simulink model "innerControllerTuning4"  (R2018a)
settings: Solver=VariableStepAuto  StartTime=0.0  StopTime=10  RelTol=1e-3
values from neighbouring files (symbols this model uses):
  d = 2.4*10^-3    (= 0.0024)    [innerInit.m]    (also in outerInit.m)
  g = 9.81    [innerInit.m]    (also in outerInit.m)
  Ixx = 5.9*10^-3    (= 0.0059)    [innerInit.m]    (also in outerInit.m)
  Iyy = 5.9*10^-3    (= 0.0059)    [innerInit.m]    (also in outerInit.m)
  Izz = 1.16*10^-3    (= 0.00116)    [innerInit.m]    (also in outerInit.m)
  kr = 0.1    [innerInit.m]    (also in outerInit.m)
  kt = 0.1    [innerInit.m]    (also in outerInit.m)
  l = 0.255    [innerInit.m]    (also in outerInit.m)
  m = 0.5    [innerInit.m]    (also in outerInit.m)
  p0 = 0.5    [innerInit.m]
  phi0 = pi/4    (= 0.785398163397)    [innerInit.m]
  q0 = 0.5    [innerInit.m]
  r0 = 2.7    [innerInit.m]
  theta0 = pi/4    (= 0.785398163397)    [innerInit.m]
libraries: simulink x2, aerolibutil x1
settings Model: Creator=giuseppe  LastModifiedBy=giuseppe

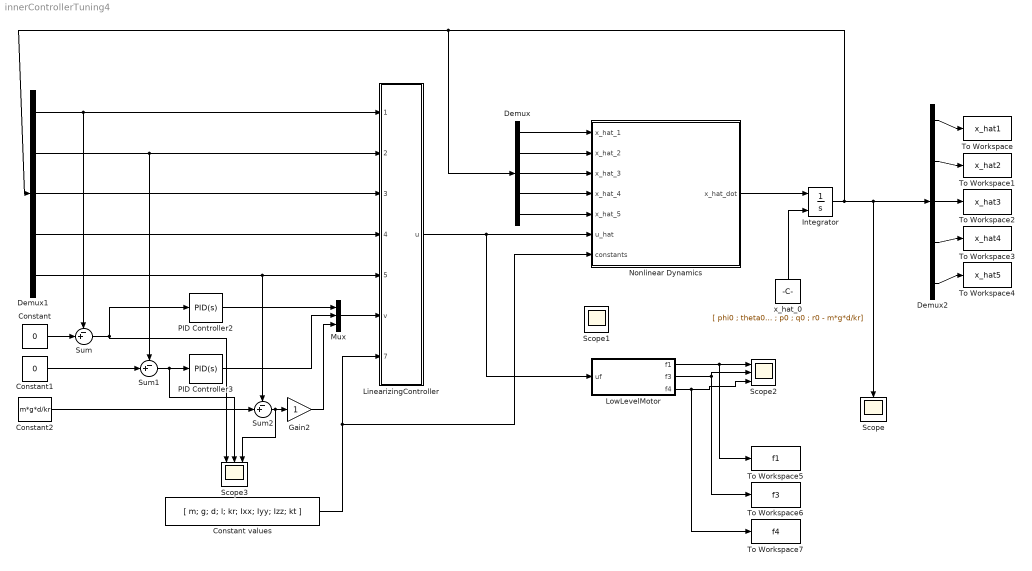
== system innerControllerTuning4 ==
  Constant : Constant  Value=0
  Constant values : Constant  Value=[ m; g; d; l; kr; Ixx; Iyy; Izz; kt ]
  Constant1 : Constant  Value=0
  Constant2 : Constant  Value=m*g*d/kr
  Demux : Demux  Outputs=5
  Demux1 : Demux  Outputs=5
  Demux2 : Demux  Outputs=5
  Gain2 : Gain
  Integrator : Integrator  InitialConditionSource=external
  LinearizingController : MATLAB Function  TreatAsAtomicUnit=on
  LowLevelMotor : Subsystem
  Mux : Mux  Inputs=3
  "Nonlinear Dynamics " : MATLAB Function  TreatAsAtomicUnit=on
  PID Controller2 : simulink/Continuous/PID Controller  Controller=PID  TimeDomain=Continuous-time  SampleTime=-1  IntegratorMethod=Forward Euler  FilterMethod=Forward Euler  Form=Parallel  UseFilter=on  ControllerParametersSource=internal  P=5  I=1  D=2  N=100  InitialConditionSource=internal  InitialConditionForIntegrator=0  InitialConditionForFilter=0  ExternalReset=none  LimitOutput=off  UpperSaturationLimit=inf  LowerSaturationLimit=-inf  LinearizeAsGain=on  AntiWindupMode=none  Kb=1  TrackingMode=off  Kt=1  PParamMin=[]  PParamMax=[]  IParamMin=[]  IParamMax=[]  DParamMin=[]  DParamMax=[]  NParamMin=[]  NParamMax=[]  KbParamMin=[]  KbParamMax=[]  KtParamMin=[]  KtParamMax=[]  POutMin=[]  POutMax=[]  IOutMin=[]  IOutMax=[]  DOutMin=[]  DOutMax=[]  NOutMin=[]  NOutMax=[]  KbOutMin=[]  KbOutMax=[]  KtOutMin=[]  KtOutMax=[]  IntegratorOutMin=[]  IntegratorOutMax=[]  FilterOutMin=[]  FilterOutMax=[]  SumOutMin=[]  SumOutMax=[]  SumI1OutMin=[]  SumI1OutMax=[]  SumI2OutMin=[]  SumI2OutMax=[]  SumI3OutMin=[]  SumI3OutMax=[]  SumDOutMin=[]  SumDOutMax=[]  SaturationOutMin=[]  SaturationOutMax=[]  IntegratorContinuousStateAttributes=''  IntegratorStateMustResolveToSignalObject=off  IntegratorRTWStateStorageClass=Auto  FilterContinuousStateAttributes=''  FilterStateMustResolveToSignalObject=off  FilterRTWStateStorageClass=Auto  DifferentiatorICPrevScaledInput=0  DifferentiatorOutMin=[]  DifferentiatorOutMax=[]  FilterDiffOutCoefMin=[]  FilterDiffOutCoefMax=[]  SumDenOutMin=[]  SumDenOutMax=[]  SumNumOutMin=[]  SumNumOutMax=[]  ReciprocalOutMin=[]  ReciprocalOutMax=[]  DivideOutMin=[]  DivideOutMax=[]  TunerSelectOption=Transfer Function Based (PID Tuner App)
  PID Controller3 : simulink/Continuous/PID Controller  Controller=PID  TimeDomain=Continuous-time  SampleTime=-1  IntegratorMethod=Forward Euler  FilterMethod=Forward Euler  Form=Parallel  UseFilter=on  ControllerParametersSource=internal  P=5  I=1  D=2  N=100  InitialConditionSource=internal  InitialConditionForIntegrator=0  InitialConditionForFilter=0  ExternalReset=none  LimitOutput=off  UpperSaturationLimit=inf  LowerSaturationLimit=-inf  LinearizeAsGain=on  AntiWindupMode=none  Kb=1  TrackingMode=off  Kt=1  PParamMin=[]  PParamMax=[]  IParamMin=[]  IParamMax=[]  DParamMin=[]  DParamMax=[]  NParamMin=[]  NParamMax=[]  KbParamMin=[]  KbParamMax=[]  KtParamMin=[]  KtParamMax=[]  POutMin=[]  POutMax=[]  IOutMin=[]  IOutMax=[]  DOutMin=[]  DOutMax=[]  NOutMin=[]  NOutMax=[]  KbOutMin=[]  KbOutMax=[]  KtOutMin=[]  KtOutMax=[]  IntegratorOutMin=[]  IntegratorOutMax=[]  FilterOutMin=[]  FilterOutMax=[]  SumOutMin=[]  SumOutMax=[]  SumI1OutMin=[]  SumI1OutMax=[]  SumI2OutMin=[]  SumI2OutMax=[]  SumI3OutMin=[]  SumI3OutMax=[]  SumDOutMin=[]  SumDOutMax=[]  SaturationOutMin=[]  SaturationOutMax=[]  IntegratorContinuousStateAttributes=''  IntegratorStateMustResolveToSignalObject=off  IntegratorRTWStateStorageClass=Auto  FilterContinuousStateAttributes=''  FilterStateMustResolveToSignalObject=off  FilterRTWStateStorageClass=Auto  DifferentiatorICPrevScaledInput=0  DifferentiatorOutMin=[]  DifferentiatorOutMax=[]  FilterDiffOutCoefMin=[]  FilterDiffOutCoefMax=[]  SumDenOutMin=[]  SumDenOutMax=[]  SumNumOutMin=[]  SumNumOutMax=[]  ReciprocalOutMin=[]  ReciprocalOutMax=[]  DivideOutMin=[]  DivideOutMax=[]  TunerSelectOption=Transfer Function Based (PID Tuner App)
  Scope : Scope
  Scope1 : Scope
  Scope2 : Scope  NumInputPorts=3
  Scope3 : Scope  NumInputPorts=3
  Sum : Sum  Inputs=-+|
  Sum1 : Sum  Inputs=-+|
  Sum2 : Sum  Inputs=-+|
  To Workspace : ToWorkspace  VariableName=x_hat1  SaveFormat=Timeseries  SampleTime=-1
  To Workspace1 : ToWorkspace  VariableName=x_hat2  SaveFormat=Timeseries  SampleTime=-1
  To Workspace2 : ToWorkspace  VariableName=x_hat3  SaveFormat=Timeseries  SampleTime=-1
  To Workspace3 : ToWorkspace  VariableName=x_hat4  SaveFormat=Timeseries  SampleTime=-1
  To Workspace4 : ToWorkspace  VariableName=x_hat5  SaveFormat=Timeseries  SampleTime=-1
  To Workspace5 : ToWorkspace  VariableName=f1  SaveFormat=Timeseries  SampleTime=-1
  To Workspace6 : ToWorkspace  VariableName=f3  SaveFormat=Timeseries  SampleTime=-1
  To Workspace7 : ToWorkspace  VariableName=f4  SaveFormat=Timeseries  SampleTime=-1
  x_hat_0 : Constant  Value=[ phi0 ; theta0 ; p0 ; q0 ; r0 - m*g*d/kr]
  wires:
  LinearizingController/1(u) -> LowLevelMotor/1(uf), "Nonlinear Dynamics "/6(u_hat)
  Constant values/1 -> "Nonlinear Dynamics "/7(constants), LinearizingController/7(constants)
  "Nonlinear Dynamics "/1(x_hat_dot) -> Integrator/1
  x_hat_0/1 -> Integrator/2
  Demux/1 -> "Nonlinear Dynamics "/1(x_hat_1)
  Demux/2 -> "Nonlinear Dynamics "/2(x_hat_2)
  Demux/3 -> "Nonlinear Dynamics "/3(x_hat_3)
  Demux/4 -> "Nonlinear Dynamics "/4(x_hat_4)
  Demux/5 -> "Nonlinear Dynamics "/5(x_hat_5)
  Integrator/1 -> Demux1/1, Demux/1, Demux2/1, Scope/1
  Demux1/5 -> LinearizingController/5(x5_hat), Sum2/1
  Demux1/4 -> LinearizingController/4(x4_hat)
  Demux1/3 -> LinearizingController/3(x3_hat)
  Demux1/2 -> Sum1/1, LinearizingController/2(x2_hat)
  Demux1/1 -> Sum/1, LinearizingController/1(x1_hat)
  Constant/1 -> Sum/2
  Constant1/1 -> Sum1/2
  Constant2/1 -> Sum2/2
  Mux/1 -> LinearizingController/6(v)
  Sum/1 -> PID Controller2/1, Scope3/1
  Sum2/1 -> Scope3/3, Gain2/1
  Gain2/1 -> Mux/3
  Sum1/1 -> PID Controller3/1, Scope3/2
  Demux2/5 -> To Workspace4/1
  Demux2/4 -> To Workspace3/1
  Demux2/3 -> To Workspace2/1
  Demux2/2 -> To Workspace1/1
  Demux2/1 -> To Workspace/1
  LowLevelMotor/3(f4) -> To Workspace7/1, Scope2/3
  LowLevelMotor/1(f1) -> To Workspace5/1, Scope2/1
  LowLevelMotor/2(f3) -> To Workspace6/1, Scope2/2
  PID Controller2/1 -> Mux/1
  PID Controller3/1 -> Mux/2

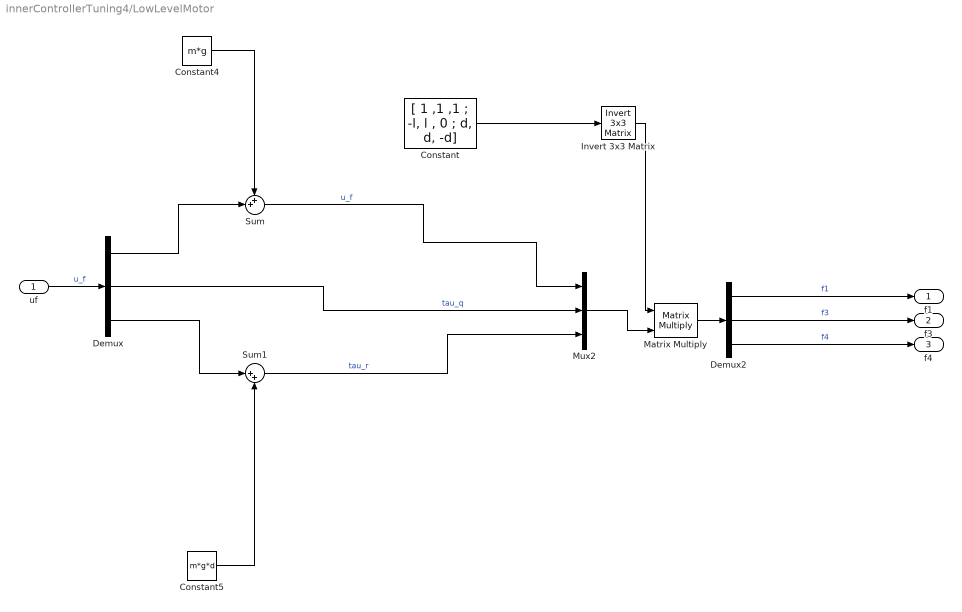
== system innerControllerTuning4/LowLevelMotor ==
  uf : Inport
  Constant : Constant  Value=[ 1 ,1 ,1 ; -l, l , 0 ; d, d, -d]
  Constant4 : Constant  Value=m*g
  Constant5 : Constant  Value=m*g*d
  Demux : Demux  Outputs=3
  Demux2 : Demux  Outputs=3
  Invert 3x3 Matrix : aerolibutil/Invert  3x3 Matrix
  Matrix Multiply : Product  Multiplication=Matrix(*)
  Mux2 : Mux  Inputs=3
  Sum : Sum  Inputs=++|
  Sum1 : Sum  Inputs=|++
  f1 : Outport
  f3 : Outport  Port=2
  f4 : Outport  Port=3
  wires:
  Demux/2 -> Mux2/2  "tau_q"
  Invert 3x3 Matrix/1 -> Matrix Multiply/1
  Sum1/1 -> Mux2/3  "tau_r"
  Mux2/1 -> Matrix Multiply/2
  Matrix Multiply/1 -> Demux2/1
  Sum/1 -> Mux2/1  "u_f"
  Constant/1 -> Invert 3x3 Matrix/1
  uf/1 -> Demux/1  "u_f"
  Constant4/1 -> Sum/1
  Demux/1 -> Sum/2
  Demux/3 -> Sum1/1
  Constant5/1 -> Sum1/2
  Demux2/1 -> f1/1  "f1"
  Demux2/2 -> f3/1  "f3"
  Demux2/3 -> f4/1  "f4"

== matlab function innerControllerTuning4/LinearizingController ==
  data: x1_hat input; u output; x2_hat input; x3_hat input; x4_hat input; x5_hat input; v input; constants input
function u = fcn(x1_hat,x2_hat,x3_hat,x4_hat,x5_hat, v, constants)

m= constants(1,1);
g= constants(2,1);
d= constants(3,1);
l= constants(4,1);
kr= constants(5,1);
Ixx= constants(6,1)
Iyy= constants(7,1);
Izz= constants(8,1);

alfa = zeros(3,1);

%% Non-robust feedback-linearation

alfa(1,1) = (2*Ixx*((kr*x3_hat - x4_hat*(x5_hat + (d*g*m)/kr)*(Ixx - Izz))/Ixx + (sin(x1_hat)*tan(x2_hat)*(x5_hat + (d*g*m)/kr) - x4_hat*cos(x1_hat)*tan(x2_hat))*(x3_hat + cos(x1_hat)*tan(x2_hat)*(x5_hat + (d*g*m)/kr) + x4_hat*sin(x1_hat)*tan(x2_hat)) + (sin(x1_hat)*(x5_hat + (d*g*m)/kr) - x4_hat*cos(x1_hat))*(cos(x1_hat)*(x5_hat + (d*g*m)/kr)*(tan(x2_hat)^2 + 1) + x4_hat*sin(x1_hat)*(tan(x2_hat)^2 + 1)) + (sin(x1_hat)*tan(x2_hat)*(kr*x4_hat + x3_hat*(x5_hat + (d*g*m)/kr)*(Ixx - Izz)))/Ixx + (kr*x5_hat*cos(x1_hat)*tan(x2_hat))/Izz))/l - (2*Ixx*sin(x1_hat)*tan(x2_hat)*((cos(x1_hat)*(x5_hat + (d*g*m)/kr) + x4_hat*sin(x1_hat))*(x3_hat + cos(x1_hat)*tan(x2_hat)*(x5_hat + (d*g*m)/kr) + x4_hat*sin(x1_hat)*tan(x2_hat)) + (cos(x1_hat)*(kr*x4_hat + x3_hat*(x5_hat + (d*g*m)/kr)*(Ixx - Izz)))/Ixx - (kr*x5_hat*sin(x1_hat))/Izz))/(l*cos(x1_hat)) - (kr*x5_hat*(2*Ixx*d*cos(x1_hat)^2*tan(x2_hat) - Izz*l*cos(x1_hat) + 2*Ixx*d*sin(x1_hat)^2*tan(x2_hat)))/(Izz*d*l*cos(x1_hat));
alfa(2,1) = (Ixx*((cos(x1_hat)*(x5_hat + (d*g*m)/kr) + x4_hat*sin(x1_hat))*(x3_hat + cos(x1_hat)*tan(x2_hat)*(x5_hat + (d*g*m)/kr) + x4_hat*sin(x1_hat)*tan(x2_hat)) + (cos(x1_hat)*(kr*x4_hat + x3_hat*(x5_hat + (d*g*m)/kr)*(Ixx - Izz)))/Ixx - (kr*x5_hat*sin(x1_hat))/Izz))/cos(x1_hat) + (Ixx*kr*x5_hat*sin(x1_hat))/(Izz*cos(x1_hat));
alfa(3,1) = kr*x5_hat;

beta =  [
         (2*Ixx)/l, -(2*Ixx*sin(x1_hat)*sin(x2_hat))/(l*cos(x1_hat)*cos(x2_hat)), -(2*Ixx*d*sin(x2_hat)-Izz*l*cos(x1_hat)*cos(x2_hat))/(d*l*cos(x1_hat)*cos(x2_hat));
         0,                                              Ixx/cos(x1_hat),                                                        (Ixx*sin(x1_hat))/cos(x1_hat);
         0,                                                            0,                                                                                  Izz];

%% Robust feedback linearization

% alfa(1,1) = x1_hat*((d*g*m*((2*Ixx*((d*g*m)/kr + (d*g*m*(Ixx - Izz))/(Ixx*kr)))/l + (2*kr*sin(x1_hat)*tan(x2_hat))/(l*cos(x1_hat))))/kr - (2*Ixx*d^2*g^2*m^2)/(kr^2*l)) - (sin(x1_hat)*(x5_hat + (d*g*m)/kr) - x4_hat*cos(x1_hat))*((2*Ixx*((d*g*m)/kr + (d*g*m*(Ixx - Izz))/(Ixx*kr)))/l + (2*kr*sin(x1_hat)*tan(x2_hat))/(l*cos(x1_hat))) + x2_hat*((d*g*m*((2*kr)/l - (2*Ixx*sin(x1_hat)*tan(x2_hat)*((d*g*m)/kr + (d*g*m*(Ixx - Izz))/(Ixx*kr)))/(l*cos(x1_hat))))/kr + (2*Ixx*d^2*g^2*m^2*sin(x1_hat)*tan(x2_hat))/(kr^2*l*cos(x1_hat))) - ((2*kr)/l - (2*Ixx*sin(x1_hat)*tan(x2_hat)*((d*g*m)/kr + (d*g*m*(Ixx - Izz))/(Ixx*kr)))/(l*cos(x1_hat)))*(x3_hat + cos(x1_hat)*tan(x2_hat)*(x5_hat + (d*g*m)/kr) + x4_hat*sin(x1_hat)*tan(x2_hat)) + (2*Ixx*((kr*x3_hat - x4_hat*(x5_hat + (d*g*m)/kr)*(Ixx - Izz))/Ixx + (sin(x1_hat)*tan(x2_hat)*(x5_hat + (d*g*m)/kr) - x4_hat*cos(x1_hat)*tan(x2_hat))*(x3_hat + cos(x1_hat)*tan(x2_hat)*(x5_hat + (d*g*m)/kr) + x4_hat*sin(x1_hat)*tan(x2_hat)) + (sin(x1_hat)*(x5_hat + (d*g*m)/kr) - x4_hat*cos(x1_hat))*(cos(x1_hat)*(x5_hat + (d*g*m)/kr)*(tan(x2_hat)^2 + 1) + x4_hat*sin(x1_hat)*(tan(x2_hat)^2 + 1)) + (sin(x1_hat)*tan(x2_hat)*(kr*x4_hat + x3_hat*(x5_hat + (d*g*m)/kr)*(Ixx - Izz)))/Ixx + (kr*x5_hat*cos(x1_hat)*tan(x2_hat))/Izz))/l - (2*Ixx*sin(x1_hat)*tan(x2_hat)*((cos(x1_hat)*(x5_hat + (d*g*m)/kr) + x4_hat*sin(x1_hat))*(x3_hat + cos(x1_hat)*tan(x2_hat)*(x5_hat + (d*g*m)/kr) + x4_hat*sin(x1_hat)*tan(x2_hat)) + (cos(x1_hat)*(kr*x4_hat + x3_hat*(x5_hat + (d*g*m)/kr)*(Ixx - Izz)))/Ixx - (kr*x5_hat*sin(x1_hat))/Izz))/(l*cos(x1_hat));
% alfa(2,1) = (kr*x5_hat*sin(x1_hat) - kr*x4_hat*cos(x1_hat) + d*g*m*sin(x1_hat))/cos(x1_hat) + (Ixx*((cos(x1_hat)*(kr*x4_hat + (x3_hat*(kr*x5_hat + d*g*m)*(Ixx - Izz))/kr))/Ixx + ((kr*x5_hat*cos(x1_hat) + kr*x4_hat*sin(x1_hat) + d*g*m*cos(x1_hat))*(x3_hat + x4_hat*sin(x1_hat)*tan(x2_hat) + (cos(x1_hat)*tan(x2_hat)*(kr*x5_hat + d*g*m))/kr))/kr - (kr*x5_hat*sin(x1_hat))/Izz))/cos(x1_hat) - (d*g*m*x1_hat)/cos(x1_hat) - (d*g*m*(2*Ixx - Izz)*(x3_hat + x4_hat*sin(x1_hat)*tan(x2_hat) + (cos(x1_hat)*tan(x2_hat)*(kr*x5_hat + d*g*m))/kr))/(kr*cos(x1_hat)) + (d^2*g^2*m^2*x2_hat*(Ixx - Izz))/(kr^2*cos(x1_hat));
% alfa(3,1) = 0;
% 
% beta = [
%         1, -(2*sin(x1_hat)*sin(x2_hat))/(l*cos(x1_hat)*cos(x2_hat)), -(2*Ixx*sin(x2_hat))/(Izz*l*cos(x1_hat)*cos(x2_hat));
%         0,                                            1/cos(x1_hat),                  (Ixx*sin(x1_hat))/(Izz*cos(x1_hat));
%         0,                                                        0,                                                    1];
    
u = alfa + beta*v;

== matlab function innerControllerTuning4/Nonlinear Dynamics  ==
  data: x_hat_1 input; x_hat_2 input; x_hat_3 input; x_hat_4 input; x_hat_5 input; x_hat_dot output; u_hat input; constants input
function x_hat_dot = fcn(x_hat_1,x_hat_2,x_hat_3,x_hat_4,x_hat_5,u_hat,constants)

m= constants(1,1);
g= constants(2,1);
d= constants(3,1);
l= constants(4,1);
kr= constants(5,1);
Ixx= constants(6,1);
Iyy= constants(7,1);
Izz= constants(8,1);

x_hat = [x_hat_1;
        x_hat_2;
        x_hat_3;
        x_hat_4;
        x_hat_5];

f = [
    x_hat(3,1)+x_hat(4,1)*sin(x_hat(1,1))*tan(x_hat(2,1)) + ( x_hat(5,1)+ m*g*d/kr)*cos(x_hat(1,1))*tan(x_hat(2,1));
    x_hat(4,1)*cos(x_hat(1,1)) - (x_hat(5,1)+ m*g*d/kr)*sin(x_hat(1,1)) ;
    1/Ixx*( -kr*x_hat(3,1) - x_hat(4,1)*(x_hat(5,1)+ m*g*d/kr)*(Izz - Ixx));
    1/Iyy*( -kr*x_hat(4,1) - x_hat(3,1)*(x_hat(5,1)+ m*g*d/kr)*(Ixx - Izz));
    1/Izz*( -kr*x_hat(5,1));    
    ];
G = [
    0 , 0 , 0;
    0,  0 , 0;
    l/(2*Ixx), 0 , -l/(2*d*Ixx)
    0,  1/Iyy  , 0 ;
    0 ,  0   ,  1/Izz;
    ];

    
x_hat_dot = f + G*u_hat;
